simulink model "direct_RFOC_hystresis_controllerME"  (R2021a)
settings: Solver=FixedStepAuto  StartTime=0.0  StopTime=10  FixedStep=1e-6  MaxStep=10e-6  RelTol=1e-3
values from neighbouring files (symbols this model uses):
  Delta = 0.1    [ParametersIM.m]    (also in parameters.m)
  Llr = 0.005839    [ParametersIM.m]    (also in parameters.m)
  Lls = 0.005839    [ParametersIM.m]    (also in parameters.m)
  Lm = 0.1722    [ParametersIM.m]    (also in parameters.m)
  Lr = Llr+Lm    (= 0.178039)    [ParametersIM.m]    (also in parameters.m)
  P = 4    [ParametersIM.m]    (also in parameters.m)
  Rotor_Flux = .9    (= 0.9)    [ParametersIM.m]    (also in parameters.m)
  Rs = 1.405    [ParametersIM.m]    (also in parameters.m)
  Taur = Lr/rr    (= 0.127626523297)    [parameters.m]
libraries: spsIGBTDiodeLib x6, spsVoltageMeasurementLib x3, spsGroundLib x2, pid_lib x2, eeStairGenerator x2, spsabctodq0Lib x2, spsDCVoltageSourceLib x1, spsdq0toabcLib x1, spsAsynchronousMachineSIUnitsLib x1, spspowerguiLib x1
settings Model: SimulationMode=accelerator  Creator=Osama  LastModifiedBy=User
settings SolverCC: AlgebraicLoopSolver=TrustRegion
settings DataIOCC: SaveFormat=StructureWithTime
settings OptimizationCC: LifeSpan=inf
settings DebuggingCC: SFExecutionAtInitializationDiag=none  SFMachineParentedDataDiag=warning  ArithmeticOperatorsInVariantConditions=warning
settings HardwareCC: ProdBitPerSizeT=32  ProdBitPerPtrDiffT=32  ProdWordSize=32  ProdHWDeviceType=Specified
settings SFSimCC: CustomCodeUndefinedFunction=UseInterfaceOnly
settings CodeAppCC: StateflowObjectComments=on
settings SimscapeCC: SimscapeNormalizeSystem=off

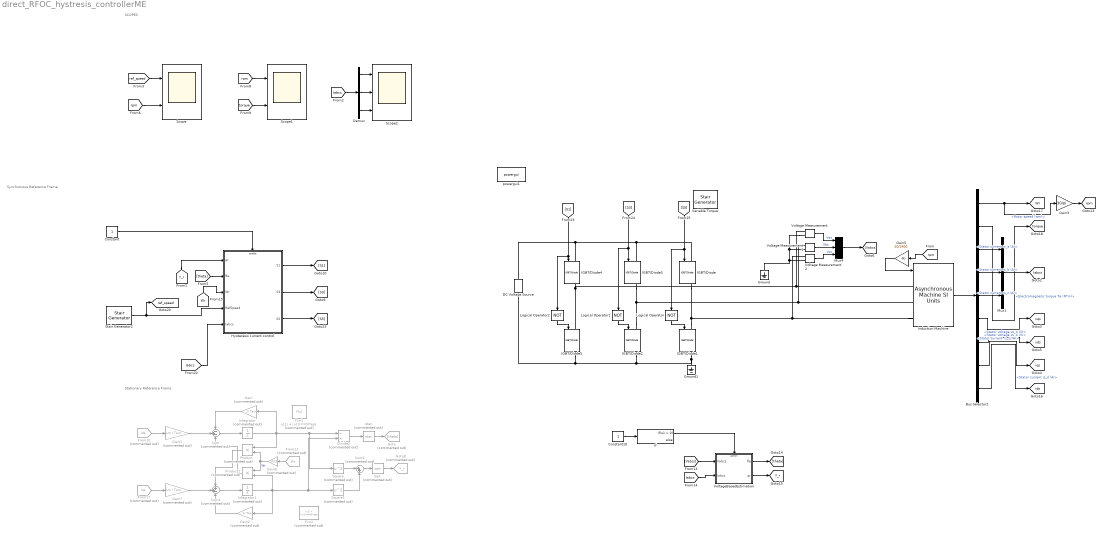
== system direct_RFOC_hystresis_controllerME ==
  note: Synchronous Reference Frame
  note: Stationary Reference Frame
  note: SCOPES
  Atan : Trigonometry  Commented=on  Operator=atan
  Bus Selector2 : BusSelector  OutputSignals="Mechanical.Rotor speed (wm),Mechanical.Electromagnetic torque Te (N*m),Stator measurements.Stator current is_a (A),Stator measurements.Stator current is_b (A),Stator measurements.Stator current is_c (A),Stator measurements.Stator voltage vs_q (V),Stator measurements.Stator voltage vs_d (V),Stator measurements.Stator current  is_q (A),Stator measurements.Stator current is_d (A)"
  Constant : Constant
  Constant10 : Constant
  DC Voltage Source : spsDCVoltageSourceLib/DC Voltage Source  Amplitude=650  Measurements=None
  Demux : Demux  Outputs=3
  Divide1 : Product  Commented=on  Inputs=/*
  Fcn1 : Fcn  Commented=on  Expr=u(1) + (u(1)==0)*eps
  Fcn2 : Fcn  Commented=on  Expr=u(1) + (u(1)==0)*eps
  From10 : From  Commented=on  GotoTag=ids  TagVisibility=global
  From12 : From  Commented=on  GotoTag=Wr  TagVisibility=global
  From17 : From  Commented=on  GotoTag=iqs  TagVisibility=global
  Gain : Gain  Commented=on  Gain=1/ Taur
  Gain1 : Gain  Commented=on  Gain=Lm / Taur
  Gain2 : Gain  Commented=on  Gain=1/ Taur
  Gain3 : Gain  Gain=30/pi
  Gain5 : Gain  Gain=20/1400
  Gain7 : Gain  Commented=on  Gain=Lm / Taur
  Gain8 : Gain  Commented=on  Gain=P/2
  Goto : Goto  Commented=on  GotoTag=theta
  Goto8 : Goto  Commented=on  GotoTag=Y_r  TagVisibility=global
  Ground : spsGroundLib/Ground  LConnTagsString=a
  Ground1 : spsGroundLib/Ground  LConnTagsString=a
  Hysteresis current control : Subsystem
  IGBT/Diode{,1..5} (6 alike) : spsIGBTDiodeLib/IGBT//Diode  Ron=1e-3  Rs=1e5  Cs=inf  Measurements=on
  If : If
  Induction Machine : spsAsynchronousMachineSIUnitsLib/Asynchronous Machine SI Units  RotorType=Squirrel-cage  PresetModel="15:  5.4 HP (4KW)   400 V  50Hz 1430 RPM"  MechanicalLoad=Torque Tm  ShowDetailedParameters=on  ReferenceFrame=Stationary  Units=SI  MeasurementBus=off  NominalParameters=[4000 400 50]  VoltageRatio=1  Stator=[1.405 0.005839]  Rotor=[1.395 0.005839]  Cage1=[0.4155 0.002066]  Cage2=[0.4168 0.0003495]  Lm=0.1722  Mechanical=[0.0131 0.002985 2]  PolePairs=2  InitialConditions=[1 0 0 0 0 0 0 0]  SimulateSaturation=off  Saturation=[14.03593122, 27.81365428, 53.79336849, 72.68890987, 97.98006896, 148.6815601, 215.7428561, 302.9841135, 428.7778367 ; 230, 322, 414, 460, 506, 552, 598, 644, 690]  LoadFlowParameters=1492000  TsPowergui=0  TsBlock=-1  IterativeModel=Trapezoidal non iterative  IterativeDiscreteModel=Trapezoidal non iterative  Pmec=1.492e+006
  Integrator : Integrator  Commented=on
  Integrator1 : Integrator  Commented=on
  Logical Operator : Logic  Operator=NOT  AllPortsSameDT=off  OutDataTypeStr=boolean
  Logical Operator1 : Logic  Operator=NOT  AllPortsSameDT=off  OutDataTypeStr=boolean
  Logical Operator2 : Logic  Operator=NOT  AllPortsSameDT=off  OutDataTypeStr=boolean
  Mux1 : Mux  Inputs=3
  Mux4 : Mux  Inputs=3
      settings: DisplayOption=signals
  Product : Product  Commented=on
  Product1 : Product  Commented=on
  Scope : Scope  NumInputPorts=2
  Scope1 : Scope  NumInputPorts=2
  Scope2 : Scope  NumInputPorts=3
  Sqrt : Sqrt  Commented=on  SaturateOnIntegerOverflow=on
  Square : Math  Commented=on  Operator=square  SaturateOnIntegerOverflow=on
  Square1 : Math  Commented=on  Operator=square  SaturateOnIntegerOverflow=on
  Stair Generator2 : eeStairGenerator/Stair Generator  LabelModeActiveChoice=Continuous  TimeInput="[0  2 4 6 8 10]"  AmplitudeInput=[1400 1000 1200 800 1000 1000]  SampleTime=0  RepeatPattern=off  OutDataTypeStr=double
      settings: SourceProductBaseCode=PS
  Sum : Sum  Commented=on  Inputs=-+-
  Sum3 : Sum  Commented=on  Inputs=++-
  Sum4 : Sum  Commented=on  Inputs=|++
  Variable Torque : eeStairGenerator/Stair Generator  LabelModeActiveChoice=Continuous  TimeInput=[0 1 3 5 7 9]  AmplitudeInput=[0 5 10 7.5 26 15]  SampleTime=0  RepeatPattern=off  OutDataTypeStr=double
      settings: SourceProductBaseCode=PS
  Voltage Measurement : spsVoltageMeasurementLib/Voltage Measurement  PhasorSimulation=off  OutputType=Complex  PSBequivalent=0
  Voltage Measurement1 : spsVoltageMeasurementLib/Voltage Measurement  PhasorSimulation=off  OutputType=Complex  PSBequivalent=0
  Voltage Measurement2 : spsVoltageMeasurementLib/Voltage Measurement  PhasorSimulation=off  OutputType=Complex  PSBequivalent=0
  VoltageBasedEstimation : Subsystem  TreatAsAtomicUnit=on
  powergui1 : spspowerguiLib/powergui  Priority=1  SimulationMode=Continuous  SampleTime=2e-6  frequency=60  Iterations=50  frequencyindice=0  Pbase=100e6  ErrMax=1e-4  UnitsV=kV  UnitsW=MW  buscounter=0  FunctionMessages=off  echomessages=off  EnableUseOfTLC=off  CurrentSourceSwitches=off  DisableSnubberDevices=off  DisableRonSwitches=off  DisableVfSwitches=off  DisplayEquations=off  AutomaticDiscreteSolvers=off  SolverType=Tustin/Backward Euler (TBE)  Interpol=off  ExternalGateDelay=off  methode=off  Ts=100  x0status=blocks  SPID=on  SwTol=0  HookPort=off  NonlinearTolerance=1e-4  nMaxIteration=100  ContinueOnMaxIteration=off  RestoreLinks=warning  ResistiveCurrentMeasurement=off  Frange=[0:2:500]  Ylog=off  Xlog=on  ShowGrid=off  save=off  variable=ZData  structure=0  ZoomFFT=off  StartTime=0.0  cycles=1  DisplayStyle=1  fundamental=60  FreqAxis=off  MaxFrequency=1000  frequencyindicesteady=1  RmsSteady=1  display=off
  tag scope: Iabcs=global, Wr=global, Y_r=global, ids=global, iqs=global, ref_speed=global, rpm=global, torque=global, vds=global, vqs=global
  wires:
  [ref_speed] -> Scope/1
  [rpm] -> Scope/2
  [rpm] -> Scope1/1
  [torque] -> Scope1/2
  Induction Machine/1 -> Bus Selector2/1
  Bus Selector2/2 -> [torque]  "<Electromagnetic torque Te (N*m)>"
  Bus Selector2/1 -> Gain3/1, [Wr]  "<Rotor speed (wm)>"
  Gain5/1 -> Induction Machine/1
  Bus Selector2/7 -> [vds]  "<Stator voltage vs_d (V)>"
  Bus Selector2/8 -> [iqs]  "<Stator current  is_q (A)>"
  Bus Selector2/6 -> [vqs]  "<Stator voltage vs_q (V)>"
  Bus Selector2/9 -> [ids]  "<Stator current is_d (A)>"
  Gain3/1 -> [rpm]
  Bus Selector2/3 -> Mux1/1  "<Stator current is_a (A)>"
  Bus Selector2/4 -> Mux1/2  "<Stator current is_b (A)>"
  Bus Selector2/5 -> Mux1/3  "<Stator current is_c (A)>"
  Mux1/1 -> [Iabcs]
  [rpm] -> Gain5/1
  Demux/1 -> Scope2/1
  Demux/2 -> Scope2/2
  Demux/3 -> Scope2/3
  [Iabcs] -> Demux/1
  Integrator/1 -> Square/1, Divide1/1, Product/1, Gain/1
  Integrator1/1 -> Product1/2, Divide1/2, Square1/1, Gain2/1
  Sum3/1 -> Integrator1/1
  Product1/1 -> Sum/3
  Gain1/1 -> Sum/2
  Gain7/1 -> Sum3/2
  Gain/1 -> Sum/1
  From12/1 -> Gain8/1
  Product/1 -> Sum3/1
  Gain2/1 -> Sum3/3
  Sum/1 -> Integrator/1
  From17/1 -> Gain7/1
  From10/1 -> Gain1/1
  Square/1 -> Sum4/1
  Square1/1 -> Sum4/2
  Sum4/1 -> Sqrt/1
  Sqrt/1 -> Goto8/1
  Divide1/1 -> Atan/1
  Atan/1 -> Goto/1
  Gain8/1 -> Product/2, Product1/1  "Wr"
  Logical Operator1/1 -> IGBT/Diode2/1
  Logical Operator/1 -> IGBT/Diode1/1
  Logical Operator2/1 -> IGBT/Diode5/1
  [Y_r] -> Hysteresis current control/1(ψr)
  [theta] -> Hysteresis current control/2(θe)
  [Wr] -> Hysteresis current control/3(Wr)
  Stair Generator2/1 -> [ref_speed], Hysteresis current control/4(RefSpeed)
  [Iabcs] -> Hysteresis current control/5(Iabcs)
  Hysteresis current control/1(S1) -> [S1]
  Hysteresis current control/3(S5) -> [S5]
  Hysteresis current control/2(S3) -> [S3]
  [S1] -> Logical Operator2/1, IGBT/Diode4/1
  [S3] -> Logical Operator1/1, IGBT/Diode3/1
  [S5] -> Logical Operator/1, IGBT/Diode/1
  Constant/1 -> Hysteresis current control/Enable
  Voltage Measurement2/1 -> Mux4/3  "Vcs"
  Voltage Measurement1/1 -> Mux4/2  "Vbs"
  Voltage Measurement/1 -> Mux4/1  "Vas"
  Mux4/1 -> [Vabcs]
  [Vabcs] -> VoltageBasedEstimation/1(Vabcs)
  [Iabcs] -> VoltageBasedEstimation/2(Iabcs)
  VoltageBasedEstimation/1(θe) -> [theta]
  VoltageBasedEstimation/2(ψr) -> [Y_r]
  If/1 -> VoltageBasedEstimation/Action
  Constant10/1 -> If/1
  connections:
  IGBT/Diode1/LConn1 -- Induction Machine/LConn3 -- Voltage Measurement2/LConn1 -- IGBT/Diode/RConn1
  IGBT/Diode2/LConn1 -- IGBT/Diode3/RConn1 -- Voltage Measurement1/LConn1 -- Induction Machine/LConn2
  IGBT/Diode4/RConn1 -- IGBT/Diode5/LConn1 -- Voltage Measurement/LConn1 -- Induction Machine/LConn1
  DC Voltage Source/LConn1 -- Ground1/LConn1 -- IGBT/Diode1/RConn1 -- IGBT/Diode2/RConn1 -- IGBT/Diode5/RConn1
  IGBT/Diode/LConn1 -- IGBT/Diode3/LConn1 -- IGBT/Diode4/LConn1 -- DC Voltage Source/RConn1
  Voltage Measurement/LConn2 -- Ground/LConn1 -- Voltage Measurement2/LConn2 -- Voltage Measurement1/LConn2

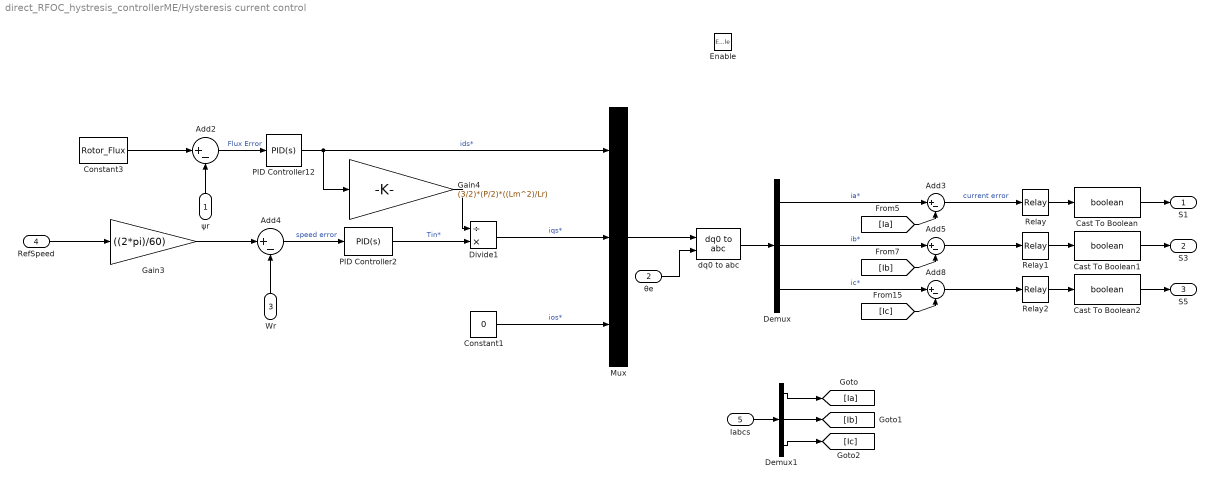
== system direct_RFOC_hystresis_controllerME/Hysteresis current control ==
  ψr : Inport
  θe : Inport  Port=2
  Wr : Inport  Port=3
  RefSpeed : Inport  Port=4
  Iabcs : Inport  Port=5
  Enable : EnablePort
  Add{2,4..5,8} (4 alike) : Sum  Inputs=|+-
  Add3 : Sum  Inputs=|+-  OutDataTypeStr=double
  Cast To Boolean : DataTypeConversion  OutDataTypeStr=boolean
  Cast To Boolean1 : DataTypeConversion  OutDataTypeStr=boolean
  Cast To Boolean2 : DataTypeConversion  OutDataTypeStr=boolean
  Constant1 : Constant  Value=0
  Constant3 : Constant  Value=Rotor_Flux
  Demux : Demux  Outputs=3
  Demux1 : Demux  Outputs=3
  Divide1 : Product  Inputs=/*
  Gain3 : Gain  Gain=((2*pi)/60)
  Gain4 : Gain  Gain=(3/2)*(P/2)*((Lm^2)/Lr)
  Mux : Mux  Inputs=3
      settings: DisplayOption=signals
  PID Controller12 : pid_lib/PID Controller  Controller=PID  Form=Parallel  TimeDomain=Continuous-time  UseExternalTs=off  SampleTime=-1  IntegratorMethod=Forward Euler  FilterMethod=Forward Euler  ControllerParametersSource=internal  P=15  I=125  D=0  UseFilter=on  N=100  TunerSelectOption=Transfer Function Based (PID Tuner App)  InitialConditionSource=internal  InitialConditionForIntegrator=0  InitialConditionForFilter=0  DifferentiatorICPrevScaledInput=0  ExternalReset=none  TrackingMode=off  Kt=1  LimitOutput=off  SatLimitsSource=internal  UpperSaturationLimit=inf  LowerSaturationLimit=-inf  LinearizeAsGain=on  AntiWindupMode=none  Kb=1  POutMin=[]  POutMax=[]  IOutMin=[]  IOutMax=[]  DOutMin=[]  DOutMax=[]  NOutMin=[]  NOutMax=[]  SumOutMin=[]  SumOutMax=[]  SaturationOutMin=[]  SaturationOutMax=[]  PParamMin=[]  PParamMax=[]  IParamMin=[]  IParamMax=[]  DParamMin=[]  DParamMax=[]  NParamMin=[]  NParamMax=[]  KbParamMin=[]  KbParamMax=[]  KtParamMin=[]  KtParamMax=[]  KbOutMin=[]  KbOutMax=[]  KtOutMin=[]  KtOutMax=[]  IntegratorOutMin=[]  IntegratorOutMax=[]  FilterOutMin=[]  FilterOutMax=[]  SumI1OutMin=[]  SumI1OutMax=[]  SumI2OutMin=[]  SumI2OutMax=[]  SumI3OutMin=[]  SumI3OutMax=[]  SumI4OutMin=[]  SumI4OutMax=[]  SumDOutMin=[]  SumDOutMax=[]  DifferentiatorOutMin=[]  DifferentiatorOutMax=[]  FilterDiffOutCoefMin=[]  FilterDiffOutCoefMax=[]  ReciprocalOutMin=[]  ReciprocalOutMax=[]  SumDenOutMin=[]  SumDenOutMax=[]  SumNumOutMin=[]  SumNumOutMax=[]  DivideOutMin=[]  DivideOutMax=[]  UdiffTsProdOutMin=[]  UdiffTsProdOutMax=[]  NTsProdOutMin=[]  NTsProdOutMax=[]  UintegralTsProdOutMin=[]  UintegralTsProdOutMax=[]  UngainTsProdOutMin=[]  UngainTsProdOutMax=[]  IntegratorContinuousStateAttributes=''  IntegratorStateMustResolveToSignalObject=off  IntegratorRTWStateStorageClass=Auto  FilterContinuousStateAttributes=''  FilterStateMustResolveToSignalObject=off  FilterRTWStateStorageClass=Auto  ParallelPVariant=InternalParameters  IdealPVariant=Disabled  IVariant=InternalParameters  DVariant=InternalParameters  IntegratorVariant=Continuous  SatVariant=Disabled  AWVariant=Passthrough  PCopyVariant=Disabled  TRVariant=Disabled  FdbkBlocksVariant=Forward  IdealPFdbkVariant=Disabled  SatFdbkVariant=Disabled  DerivativeFilterVariant=ContFilter  NVariant=InternalParameters  NCopyVariant=Disabled  FilterICVariant=InternalICsFilter  IntegratorICVariant=InternalICs  ExternalResetVariant=Disabled  TRSumVariant=Passthrough  SumFdbkVariant=Disabled  SumVariant=Sum_PID  TsampFilterVariant=InternalTs  TsampNgainVariant=Passthrough  TsampIntegralVariant=Passthrough  ExternalSaturationOutDataTypeStr=Inherit: Same as second input
  PID Controller2 : pid_lib/PID Controller  Controller=PID  Form=Parallel  TimeDomain=Continuous-time  UseExternalTs=off  SampleTime=-1  IntegratorMethod=Forward Euler  FilterMethod=Forward Euler  ControllerParametersSource=internal  P=20  I=200  D=0.1  UseFilter=on  N=100  TunerSelectOption=Transfer Function Based (PID Tuner App)  InitialConditionSource=internal  InitialConditionForIntegrator=0  InitialConditionForFilter=0  DifferentiatorICPrevScaledInput=0  ExternalReset=none  TrackingMode=off  Kt=1  LimitOutput=on  SatLimitsSource=internal  UpperSaturationLimit=100  LowerSaturationLimit=-100  LinearizeAsGain=on  AntiWindupMode=clamping  Kb=1  POutMin=[]  POutMax=[]  IOutMin=[]  IOutMax=[]  DOutMin=[]  DOutMax=[]  NOutMin=[]  NOutMax=[]  SumOutMin=[]  SumOutMax=[]  SaturationOutMin=[]  SaturationOutMax=[]  PParamMin=[]  PParamMax=[]  IParamMin=[]  IParamMax=[]  DParamMin=[]  DParamMax=[]  NParamMin=[]  NParamMax=[]  KbParamMin=[]  KbParamMax=[]  KtParamMin=[]  KtParamMax=[]  KbOutMin=[]  KbOutMax=[]  KtOutMin=[]  KtOutMax=[]  IntegratorOutMin=[]  IntegratorOutMax=[]  FilterOutMin=[]  FilterOutMax=[]  SumI1OutMin=[]  SumI1OutMax=[]  SumI2OutMin=[]  SumI2OutMax=[]  SumI3OutMin=[]  SumI3OutMax=[]  SumI4OutMin=[]  SumI4OutMax=[]  SumDOutMin=[]  SumDOutMax=[]  DifferentiatorOutMin=[]  DifferentiatorOutMax=[]  FilterDiffOutCoefMin=[]  FilterDiffOutCoefMax=[]  ReciprocalOutMin=[]  ReciprocalOutMax=[]  SumDenOutMin=[]  SumDenOutMax=[]  SumNumOutMin=[]  SumNumOutMax=[]  DivideOutMin=[]  DivideOutMax=[]  UdiffTsProdOutMin=[]  UdiffTsProdOutMax=[]  NTsProdOutMin=[]  NTsProdOutMax=[]  UintegralTsProdOutMin=[]  UintegralTsProdOutMax=[]  UngainTsProdOutMin=[]  UngainTsProdOutMax=[]  IntegratorContinuousStateAttributes=''  IntegratorStateMustResolveToSignalObject=off  IntegratorRTWStateStorageClass=Auto  FilterContinuousStateAttributes=''  FilterStateMustResolveToSignalObject=off  FilterRTWStateStorageClass=Auto  ParallelPVariant=InternalParameters  IdealPVariant=Disabled  IVariant=InternalParameters  DVariant=InternalParameters  IntegratorVariant=Continuous  SatVariant=Enabled  AWVariant=ContClampingParallel  PCopyVariant=Disabled  TRVariant=Disabled  FdbkBlocksVariant=Forward  IdealPFdbkVariant=Disabled  SatFdbkVariant=Disabled  DerivativeFilterVariant=ContFilter  NVariant=InternalParameters  NCopyVariant=Disabled  FilterICVariant=InternalICsFilter  IntegratorICVariant=InternalICs  ExternalResetVariant=Disabled  TRSumVariant=Passthrough  SumFdbkVariant=Disabled  SumVariant=Sum_PID  TsampFilterVariant=InternalTs  TsampNgainVariant=Passthrough  TsampIntegralVariant=Passthrough  ExternalSaturationOutDataTypeStr=Inherit: Same as second input
  Relay : Relay  OnSwitchValue=Delta/2  OffSwitchValue=(-1*Delta)/2
  Relay1 : Relay  OnSwitchValue=Delta/2  OffSwitchValue=(-1*Delta)/2
  Relay2 : Relay  OnSwitchValue=Delta/2  OffSwitchValue=(-1*Delta)/2
  dq0 to abc : spsdq0toabcLib/dq0 to abc  Alignment=90 degrees behind phase A axis
  S1 : Outport
  S3 : Outport  Port=2
  S5 : Outport  Port=3
  wires:
  Divide1/1 -> Mux/2  "iqs*"
  θe/1 -> dq0 to abc/2
  Demux/2 -> Add5/1  "ib*"
  PID Controller2/1 -> Divide1/2  "Tin*"
  Wr/1 -> Add4/2
  PID Controller12/1 -> Gain4/1, Mux/1  "ids*"
  RefSpeed/1 -> Gain3/1
  Mux/1 -> dq0 to abc/1
  Constant3/1 -> Add2/1
  Relay2/1 -> Cast To Boolean2/1
  Gain3/1 -> Add4/1
  Add4/1 -> PID Controller2/1  "speed error"
  Demux/3 -> Add8/1  "ic*"
  Gain4/1 -> Divide1/1
  [Ia] -> Add3/2
  Add5/1 -> Relay1/1
  Relay1/1 -> Cast To Boolean1/1
  Demux/1 -> Add3/1  "ia*"
  Add8/1 -> Relay2/1
  Constant1/1 -> Mux/3  "ios*"
  [Ic] -> Add8/2
  [Ib] -> Add5/2
  Add3/1 -> Relay/1  "current error"
  dq0 to abc/1 -> Demux/1
  Add2/1 -> PID Controller12/1  "Flux Error"
  Relay/1 -> Cast To Boolean/1
  ψr/1 -> Add2/2
  Iabcs/1 -> Demux1/1
  Demux1/1 -> [Ia]
  Demux1/2 -> [Ib]
  Demux1/3 -> [Ic]
  Cast To Boolean/1 -> S1/1
  Cast To Boolean1/1 -> S3/1
  Cast To Boolean2/1 -> S5/1

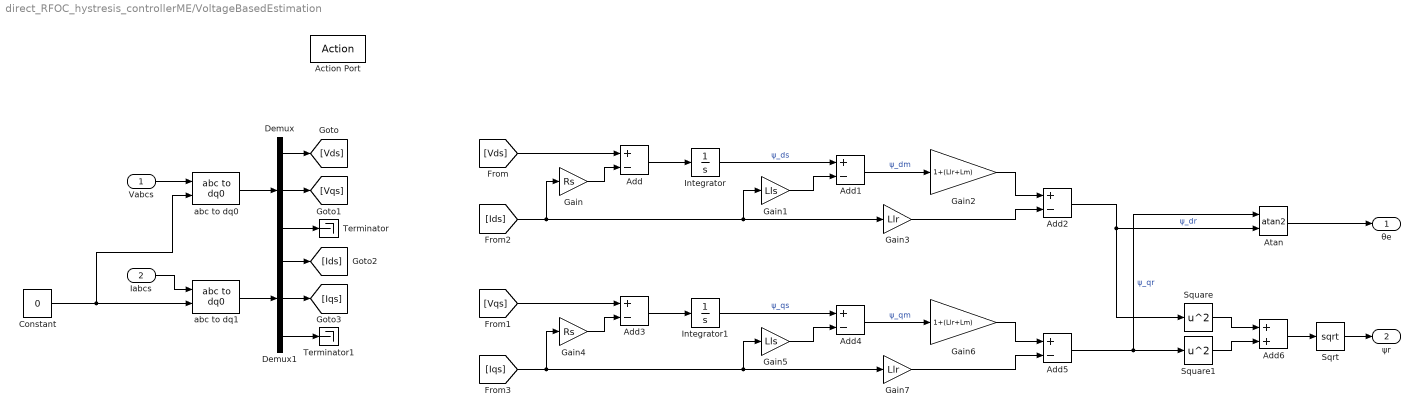
== system direct_RFOC_hystresis_controllerME/VoltageBasedEstimation ==
  Vabcs : Inport
  Iabcs : Inport  Port=2
  Action Port : ActionPort  ActionPortLabel=if(u1 > 0)
  Add{,1..5} (6 alike) : Sum  Inputs=+-
  Add6 : Sum
  Atan : Trigonometry  Operator=atan2
  Constant : Constant  Value=0
  Demux : Demux  Outputs=3
  Demux1 : Demux  Outputs=3
  Gain : Gain  Gain=Rs
  Gain1 : Gain  Gain=Lls
  Gain2 : Gain  Gain=1+(Llr+Lm)
  Gain3 : Gain  Gain=Llr
  Gain4 : Gain  Gain=Rs
  Gain5 : Gain  Gain=Lls
  Gain6 : Gain  Gain=1+(Llr+Lm)
  Gain7 : Gain  Gain=Llr
  Integrator : Integrator
  Integrator1 : Integrator
  Sqrt : Sqrt  SaturateOnIntegerOverflow=on
  Square : Math  Operator=square  SaturateOnIntegerOverflow=on
  Square1 : Math  Operator=square  SaturateOnIntegerOverflow=on
  Terminator : Terminator
  Terminator1 : Terminator
  abc to dq0 : spsabctodq0Lib/abc to dq0  Alignment=90 degrees behind phase A axis
  abc to dq1 : spsabctodq0Lib/abc to dq0  Alignment=90 degrees behind phase A axis
  θe : Outport
  ψr : Outport  Port=2
  wires:
  Vabcs/1 -> abc to dq0/1
  Iabcs/1 -> abc to dq1/1
  Constant/1 -> abc to dq0/2, abc to dq1/2
  abc to dq0/1 -> Demux/1
  Demux/1 -> [Vds]
  Demux/2 -> [Vqs]
  Demux/3 -> Terminator/1
  abc to dq1/1 -> Demux1/1
  Demux1/1 -> [Ids]
  Demux1/2 -> [Iqs]
  Demux1/3 -> Terminator1/1
  [Vds] -> Add/1
  Gain/1 -> Add/2
  [Ids] -> Gain3/1, Gain1/1, Gain/1
  Add/1 -> Integrator/1
  Integrator/1 -> Add1/1  "ψ_ds"
  Gain1/1 -> Add1/2
  Add1/1 -> Gain2/1  "ψ_dm"
  Gain2/1 -> Add2/1
  Gain3/1 -> Add2/2
  Gain7/1 -> Add5/2
  Gain6/1 -> Add5/1
  Add4/1 -> Gain6/1  "ψ_qm"
  Gain5/1 -> Add4/2
  Integrator1/1 -> Add4/1  "ψ_qs"
  Add3/1 -> Integrator1/1
  [Iqs] -> Gain4/1, Gain5/1, Gain7/1
  Gain4/1 -> Add3/2
  [Vqs] -> Add3/1
  Add2/1 -> Square/1, Atan/2  "ψ_dr"
  Add5/1 -> Atan/1, Square1/1  "ψ_qr"
  Atan/1 -> θe/1
  Square/1 -> Add6/1
  Square1/1 -> Add6/2
  Add6/1 -> Sqrt/1
  Sqrt/1 -> ψr/1
